simulink model "Week1_Q1"  (R2020b)
settings: Solver=VariableStepAuto  StartTime=0.0  StopTime=10.0  RelTol=1e-3
values from neighbouring files (symbols this model uses):
  b = 50    [Variables.m]
  k1 = 50    [Variables.m]
  k12 = 20    [Variables.m]
  M2 = 0.2    [Variables.m]
undefined symbols (not defined in the file or in its folder): M1
settings Model: Creator=vikas  LastModifiedBy=vikas

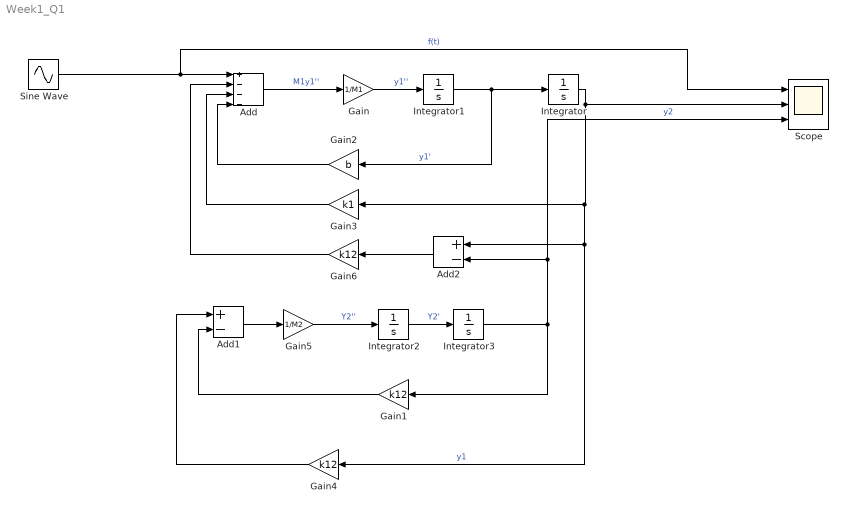
== system Week1_Q1 ==
  Add : Sum  Inputs=+---
  Add1 : Sum  Inputs=+-
  Add2 : Sum  Inputs=+-
  Gain : Gain  Gain=1/M1
  Gain1 : Gain  Gain=k12
  Gain2 : Gain  Gain=b
  Gain3 : Gain  Gain=k1
  Gain4 : Gain  Gain=k12
  Gain5 : Gain  Gain=1/M2
  Gain6 : Gain  Gain=k12
  Integrator{,1..3} (4 alike) : Integrator
  Scope : Scope  NumInputPorts=3
  Sine Wave : Sin  Amplitude=2  Frequency=10  SampleTime=0
  wires:
  Add2/1 -> Gain6/1
  Integrator1/1 -> Integrator/1, Gain2/1  "y1'"
  Sine Wave/1 -> Scope/1, Add/1  "f(t)"
  Gain2/1 -> Add/4
  Integrator2/1 -> Integrator3/1  "Y2'"
  Gain6/1 -> Add/2
  Add/1 -> Gain/1  "M1y1''"
  Integrator3/1 -> Scope/3, Add2/2, Gain1/1  "y2"
  Gain/1 -> Integrator1/1  "y1''"
  Gain5/1 -> Integrator2/1  "Y2''"
  Gain1/1 -> Add1/2
  Integrator/1 -> Add2/1, Gain4/1, Gain3/1, Scope/2  "y1"
  Gain4/1 -> Add1/1
  Add1/1 -> Gain5/1
  Gain3/1 -> Add/3
